simulink model "LongTerm_Neuron"  (R2018a)
settings: Solver=VariableStepAuto  StartTime=0.0  StopTime=86400  RelTol=1e-3
settings Model: Creator=andys  LastModifiedBy=andys

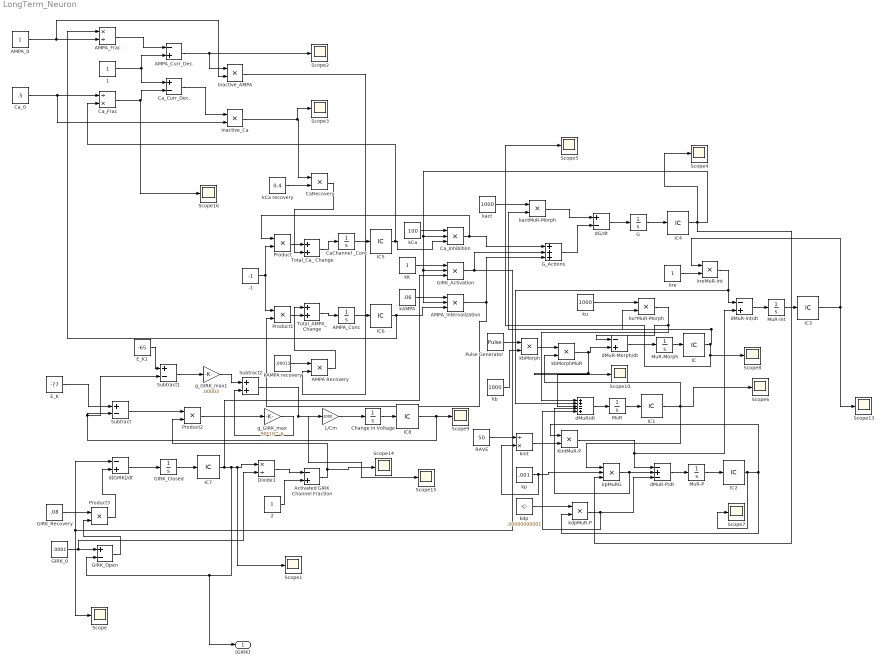
== system LongTerm_Neuron ==
  -1 : Constant  Value=-1
  1 : Constant
  1/Cm : Gain  Gain=1000
  2 : Constant
  AMPA Recovery : Product
  AMPA_0 : Constant
  AMPA_Conc : Integrator  InitialCondition=1
  AMPA_Curr_Dec. : Sum  Inputs=-+
  AMPA_Frac : Product  Inputs=*/
  AMPA_Internalization : Product  Inputs=3
  Activated GIRK Channel Fraction : Sum  Inputs=-+
  CaChannel _Conc : Integrator  InitialCondition=.5
  CaRecovery : Product
  Ca_0 : Constant  Value=.5
  Ca_Curr_Dec. : Sum  Inputs=+-
  Ca_Frac : Product  Inputs=/*
  Ca_Inhibition : Product  Inputs=3
  Change in Voltage : Integrator  InitialCondition=-65
  Divide1 : Product  Inputs=*/
  E_K : Constant  Value=-77
  E_K1 : Constant  Value=-65
  G : Integrator
  GIRK_0 : Constant  Value=.0001
  GIRK_Activation : Product  Inputs=3
  GIRK_Closed : Integrator  InitialCondition=.0001
  GIRK_Open : Sum  Inputs=+-
  GIRK_Recovery : Constant  Value=.08
  G_Actions : Sum  Inputs=+++
  IC{,2..4} (4 alike) : InitialCondition  Value=0
  IC1 : InitialCondition  Value=0.01
  IC5 : InitialCondition  Value=.5
  IC6 : InitialCondition
  IC7 : InitialCondition  Value=.0001
  IC8 : InitialCondition  Value=-65
  Inactive_AMPA : Product
  Inactive_Ca : Product
  KintMuR-P : Product
  MuR : Integrator  InitialCondition=.01
  MuR-Morph : Integrator
  MuR-P : Integrator
  MuR-int : Integrator
  Product{,1..3} (4 alike) : Product
  Pulse Generator : DiscretePulseGenerator  PulseType=Time based  Amplitude=.01  Period=100000  PulseWidth=99
  RAVE : Constant  Value=50
  Scope{,1..10,13..16} (15 alike) : Scope
  Subtract : Sum  Inputs=+-
  Subtract1 : Sum  Inputs=+-
  Subtract2 : Sum
  Total_AMPA_ Change : Sum
  Total_Ca_ Change : Sum
  dG/dt : Sum  Inputs=+-
  dMuR-Morph/dt : Sum  Inputs=-+
  dMuR-P/dt : Sum  Inputs=-+-
  dMuR-int/dt : Sum  Inputs=-+
  dMuR/dt : Sum  Inputs=++--+
  d[GIRK]/dt : Sum  Inputs=-+
  g_GIRK_max : Gain  Gain=90*10^-6
  g_GIRK_max1 : Gain  Gain=.00003
  kAMPA : Constant  Value=.06
  kAMPA recovery : Constant  Value=.00013
  kCa : Constant  Value=100
  kCa recovery : Constant  Value=0.4
  kK : Constant
  kact : Constant  Value=1000
  kactMuR-Morph : Product
  kb : Constant  Value=1000
  kbMorph : Product
  kbMorphMuR : Product
  kdp : Constant  Value=.00000000001
  kdpMuR-P : Product
  kint : Product  Inputs=/*
  kp : Constant  Value=.001
  kpMuRG : Product  Inputs=3
  kre : Constant
  kreMuR-int : Product
  ku : Constant  Value=1000
  ku*MuR-Morph : Product
  "[GIRK]" : Outport
  wires:
  g_GIRK_max/1 -> Subtract2/2
  g_GIRK_max1/1 -> Subtract2/1
  Change in Voltage/1 -> IC8/1
  Subtract1/1 -> g_GIRK_max1/1
  Ca_Inhibition/1 -> Product/1, G_Actions/1
  IC6/1 -> AMPA_Frac/1, AMPA_Internalization/3
  MuR-int/1 -> IC3/1
  AMPA_Curr_Dec./1 -> Scope2/1, Inactive_AMPA/1
  kactMuR-Morph/1 -> dG/dt/1
  kdp/1 -> kdpMuR-P/1
  dMuR/dt/1 -> MuR/1
  kre/1 -> kreMuR-int/2
  dG/dt/1 -> G/1
  Ca_Frac/1 -> Scope16/1, Ca_Curr_Dec./2
  Product1/1 -> Total_AMPA_ Change/2
  Product/1 -> Total_Ca_ Change/1
  kb/1 -> kbMorph/2
  AMPA Recovery/1 -> Total_AMPA_ Change/1
  Ca_Curr_Dec./1 -> Inactive_Ca/1
  Total_AMPA_ Change/1 -> AMPA_Conc/1
  Inactive_Ca/1 -> Scope3/1, CaRecovery/1
  Inactive_AMPA/1 -> AMPA Recovery/2
  kCa/1 -> Ca_Inhibition/1
  AMPA_Internalization/1 -> Product1/2, G_Actions/3
  CaRecovery/1 -> Total_Ca_ Change/2
  kdpMuR-P/1 -> dMuR/dt/5, dMuR-P/dt/3
  GIRK_Activation/1 -> d[GIRK]/dt/1, Scope/1, G_Actions/2
  KintMuR-P/1 -> dMuR-int/dt/2, dMuR-P/dt/1
  kCa recovery/1 -> CaRecovery/2
  IC/1 -> Scope8/1, Scope5/1, kactMuR-Morph/2, ku*MuR-Morph/2
  AMPA_0/1 -> Inactive_AMPA/2, AMPA_Frac/2
  MuR/1 -> IC1/1
  IC4/1 -> kpMuRG/3, Scope4/1, AMPA_Internalization/2, GIRK_Activation/2, Ca_Inhibition/2
  kK/1 -> GIRK_Activation/1
  kbMorphMuR/1 -> Scope10/1, dMuR/dt/3, dMuR-Morph/dt/2
  MuR-P/1 -> IC2/1
  kp/1 -> kint/2, kpMuRG/2
  dMuR-int/dt/1 -> MuR-int/1
  IC3/1 -> kreMuR-int/1, Scope13/1
  kAMPA/1 -> AMPA_Internalization/1
  G/1 -> IC4/1
  dMuR-Morph/dt/1 -> MuR-Morph/1
  kreMuR-int/1 -> dMuR/dt/2, dMuR-int/dt/1
  ku/1 -> ku*MuR-Morph/1
  IC8/1 -> Subtract1/2, Subtract/2, Scope9/1
  E_K1/1 -> Subtract1/1
  ku*MuR-Morph/1 -> dMuR-Morph/dt/1, dMuR/dt/1
  GIRK_Closed/1 -> IC7/1
  1/Cm/1 -> Change in Voltage/1
  kbMorph/1 -> kbMorphMuR/1
  Divide1/1 -> Activated GIRK Channel Fraction/1
  E_K/1 -> Subtract/1
  Product2/1 -> g_GIRK_max/1
  IC7/1 -> GIRK_Activation/3, GIRK_Open/2, "[GIRK]"/1, Scope1/1, Divide1/1
  kpMuRG/1 -> dMuR/dt/4, dMuR-P/dt/2
  CaChannel _Conc/1 -> IC5/1
  GIRK_0/1 -> Divide1/2, GIRK_Open/1
  MuR-Morph/1 -> IC/1
  IC5/1 -> Ca_Inhibition/3, Ca_Frac/2
  GIRK_Recovery/1 -> Product3/1
  Subtract/1 -> Product2/1
  Activated GIRK Channel Fraction/1 -> Scope14/1, Product2/2
  kAMPA recovery/1 -> AMPA Recovery/1
  Product3/1 -> d[GIRK]/dt/2
  1/1 -> AMPA_Curr_Dec./2, Ca_Curr_Dec./1
  d[GIRK]/dt/1 -> GIRK_Closed/1
  kact/1 -> kactMuR-Morph/1
  AMPA_Conc/1 -> IC6/1
  Pulse Generator/1 -> kbMorph/1
  -1/1 -> Product/2, Product1/1
  Ca_0/1 -> Inactive_Ca/2, Ca_Frac/1
  RAVE/1 -> kint/1
  IC1/1 -> Scope6/1, kpMuRG/1, kbMorphMuR/2
  IC2/1 -> Scope7/1, kdpMuR-P/2, KintMuR-P/1
  AMPA_Frac/1 -> AMPA_Curr_Dec./1
  G_Actions/1 -> dG/dt/2
  dMuR-P/dt/1 -> MuR-P/1
  2/1 -> Activated GIRK Channel Fraction/2
  GIRK_Open/1 -> Product3/2
  Subtract2/1 -> Scope15/1, 1/Cm/1
  kint/1 -> KintMuR-P/2
  Total_Ca_ Change/1 -> CaChannel _Conc/1
